simulink model "ClarkTran"  (R2022b)
settings: Solver=FixedStepDiscrete  StartTime=0.0  StopTime=10.0  FixedStep=0.000001  RelTol=1e-3
settings Model: Creator=yll  LastModifiedBy=yll

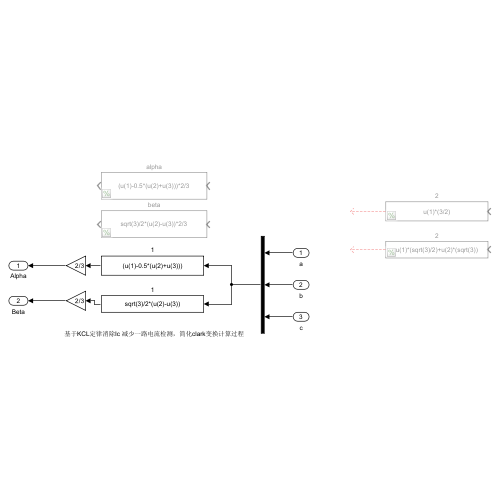
[thumbnail: Simulink's stored preview of the top-level diagram]
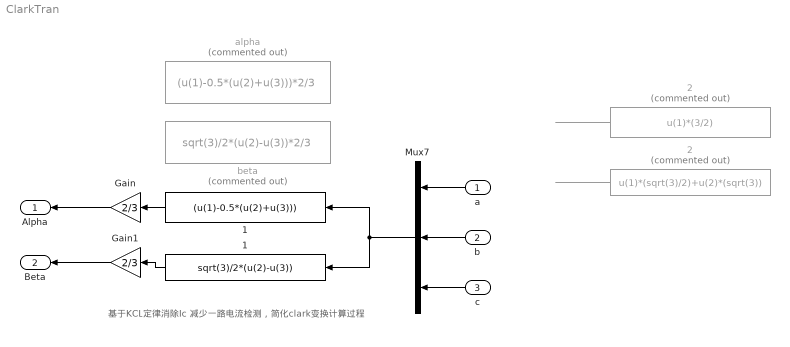
== system ClarkTran ==
  note: 基于KCL定律消除Ic 减少一路电流检测，简化clark变换计算过程
  a : Inport
  b : Inport  Port=2
  c : Inport  Port=3
  " 1" : Fcn  Expr=(u(1)-0.5*(u(2)+u(3)))
  " 2" : Fcn  Commented=on  Expr=u(1)*(3/2)
  " 1" : Fcn  Expr=sqrt(3)/2*(u(2)-u(3))
  " 2" : Fcn  Commented=on  Expr=u(1)*(sqrt(3)/2)+u(2)*(sqrt(3))
  Gain : Gain  Gain=2/3
  Gain1 : Gain  Gain=2/3
  Mux7 : Mux  Inputs=3
  alpha : Fcn  Commented=on  Expr=(u(1)-0.5*(u(2)+u(3)))*2/3
  beta : Fcn  Commented=on  Expr=sqrt(3)/2*(u(2)-u(3))*2/3
  Alpha : Outport
  Beta : Outport  Port=2
  wires:
  b/1 -> Mux7/2
  c/1 -> Mux7/3
  a/1 -> Mux7/1
  " 1"/1 -> Gain/1
  " 1"/1 -> Gain1/1
  Mux7/1 -> " 1"/1, " 1"/1
  " 2"/1 -> ?
  " 2"/1 -> ?
  Gain1/1 -> Beta/1
  Gain/1 -> Alpha/1
